simulink model "POstDeployment_ShockLoad_Calcs"  (R2022b)
settings: Solver=ode8  StartTime=0.0  StopTime=200  FixedStep=0.0001  RelTol=1e-3
values from neighbouring files (symbols this model uses):
  A_b = 0.01824    [Recovery_ShockLoad_Variables.m]
  Cdb = 0.54    [Recovery_ShockLoad_Variables.m]
  Cdp = 0.97    [Recovery_ShockLoad_Variables.m]
  g = 9.81    [Recovery_ShockLoad_Variables.m]
  mb = 38    [Recovery_ShockLoad_Variables.m]
  V_0 = 75    [Recovery_ShockLoad_Variables.m]
undefined symbols (not defined in the file or in its folder): L_m, m_m, rho, sigbuilder_block
settings Model: Creator=mohka  LastModifiedBy=mohka
settings DebuggingCC: UnconnectedInputMsg=warning  UnconnectedOutputMsg=warning  UnconnectedLineMsg=warning
settings ModelReferenceCC: EnableRefExpFcnMdlSchedulingChecks=on
settings RTWCC: DLArmComputeVersion=19.05

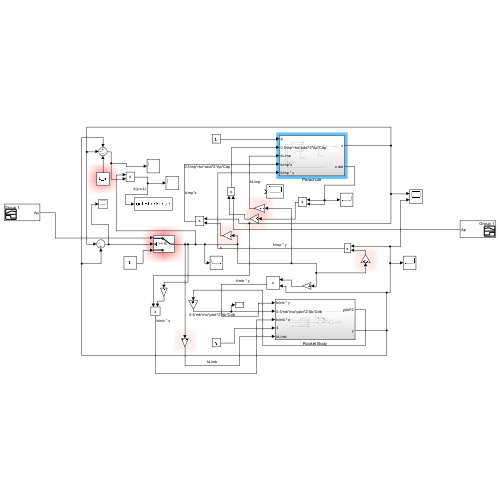
[thumbnail: Simulink's stored preview of the top-level diagram]
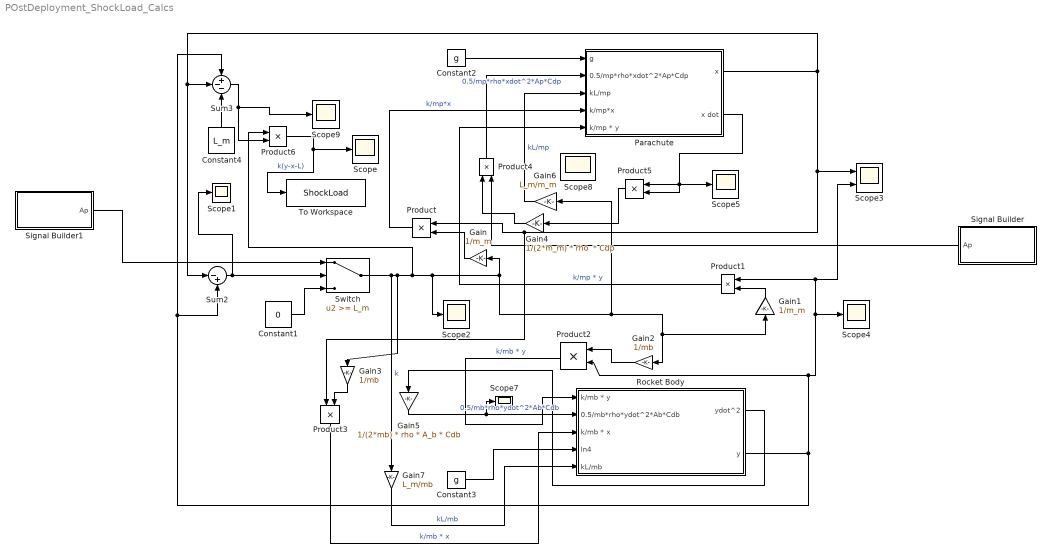
== system POstDeployment_ShockLoad_Calcs ==
  Constant1 : Constant  Value=0  VectorParams1D=off
  Constant2 : Constant  Value=g
  Constant3 : Constant  Value=g
  Constant4 : Constant  Value=L_m
  Gain : Gain  Gain=1/m_m
  Gain1 : Gain  Gain=1/m_m
  Gain2 : Gain  Gain=1/mb
  Gain3 : Gain  Gain=1/mb
  Gain4 : Gain  Gain="1/(2*m_m) * rho  * Cdp"
  Gain5 : Gain  Gain=1/(2*mb) * rho * A_b * Cdb
  Gain6 : Gain  Gain=L_m/m_m
  Gain7 : Gain  Gain=L_m/mb
  Parachute : Subsystem
  Product{,1..6} (7 alike) : Product
  Rocket Body : Subsystem
  Scope{,1..2,4..5,7..9} (8 alike) : Scope
  Scope3 : Scope  NumInputPorts=2
  Signal Builder : Subsystem  Tag=STV Subsys  LoadFcn=sigbuilder_block('load');  StartFcn=sigbuilder_block('start');  StopFcn=sigbuilder_block('stop');  ClipboardFcn=sigbuilder_block('clipboard');  mask(Sigbuilder block){tuvar=[0:10]}
      mask help: Simulink:masks:SigbuilderBlock_MD
      mask init:
      | if ~strcmp(get_param(bdroot(gcbh),'SimulationStatus'),'stopped') tuvar = sigbuilder_block('maskInit'); end
      settings: CopyFcn=sigbuilder_block('copy');  DeleteFcn=sigbuilder_block('delete');  ModelCloseFcn=sigbuilder_block('modelClose');  PreSaveFcn=sigbuilder_block('preSave');  PauseFcn=sigbuilder_block('pause');  ContinueFcn=sigbuilder_block('continue');  NameChangeFcn=sigbuilder_block('namechange');  OpenFcn=sigbuilder_block('open',[6 0 1428 711.75 ]);  CloseFcn=sigbuilder_block('close');
      mask Display: plot(0, 0, 100, 100,[2, 2, 32, 32, 2], [68, 8, 8, 68, 68],[32, 2], [38, 38], [32, 19, 2],[53, 60, 44], [32, 17, 17, 2],[16, 16, 31, 31]);txt = getActiveGroup(gcbh);text(2, 100, txt,'verticalAlignment', 'top');
  Signal Builder1 : Subsystem  Tag=STV Subsys  LoadFcn=sigbuilder_block('load');  StartFcn=sigbuilder_block('start');  StopFcn=sigbuilder_block('stop');  ClipboardFcn=sigbuilder_block('clipboard');  mask(Sigbuilder block){tuvar=[0:10]}
      mask help: Simulink:masks:SigbuilderBlock_MD
      mask init:
      | if ~strcmp(get_param(bdroot(gcbh),'SimulationStatus'),'stopped') tuvar = sigbuilder_block('maskInit'); end
      settings: CopyFcn=sigbuilder_block('copy');  DeleteFcn=sigbuilder_block('delete');  ModelCloseFcn=sigbuilder_block('modelClose');  PreSaveFcn=sigbuilder_block('preSave');  PauseFcn=sigbuilder_block('pause');  ContinueFcn=sigbuilder_block('continue');  NameChangeFcn=sigbuilder_block('namechange');  OpenFcn=sigbuilder_block('open',[116.509 88.3636 1427.56 712.145 ]);  CloseFcn=sigbuilder_block('close');
      mask Display: plot(0, 0, 100, 100,[2, 2, 32, 32, 2], [68, 8, 8, 68, 68],[32, 2], [38, 38], [32, 19, 2],[53, 60, 44], [32, 17, 17, 2],[16, 16, 31, 31]);txt = getActiveGroup(gcbh);text(2, 100, txt,'verticalAlignment', 'top');
  Sum2 : Sum  Inputs=|-+
  Sum3 : Sum  Inputs=+--
  Switch : Switch  Threshold=L_m  SaturateOnIntegerOverflow=off  InputSameDT=off
  To Workspace : ToWorkspace  VariableName=ShockLoad  SampleTime=-1
  wires:
  Gain/1 -> Product/2
  Product3/1 -> Rocket Body/3(k/mb * x)  "k/mb * x"
  Product4/1 -> Parachute/2(0.5/mp*rho*xdot^2*Ap*Cdp)  "0.5/mp*rho*xdot^2*Ap*Cdp"
  Gain7/1 -> Rocket Body/5(kL/mb)  "kL/mb"
  Product5/1 -> Gain4/1
  Rocket Body/1(ydot^2) -> Gain5/1
  Constant3/1 -> Rocket Body/4(In4)
  Constant1/1 -> Switch/3
  Parachute/2(x dot) -> Product5/1, Scope5/1, Product5/2
  Sum3/1 -> Scope9/1, Product6/2
  Product1/1 -> Parachute/5(k/mp * y)  "k/mp * y"
  Product/1 -> Parachute/4(k/mp*x)  "k/mp*x"
  Gain3/1 -> Product3/2
  Gain1/1 -> Product1/2
  Gain6/1 -> Parachute/3(kL/mp)  "kL/mp"
  Parachute/1(x) -> Product/1, Product3/1, Scope3/1, Sum2/1, Sum3/2
  Gain4/1 -> Product4/1
  Gain2/1 -> Product2/1
  Constant2/1 -> Parachute/1(g)
  Rocket Body/2(y) -> Scope3/2, Product1/1, Scope4/1, Product2/2, Sum3/1, Sum2/2
  Product6/1 -> To Workspace/1, Scope/1  "k(y-x-L)"
  Switch/1 -> Scope2/1, Gain/1, Gain6/1, Gain2/1, Gain1/1, Product6/1, Gain3/1, Gain7/1  "k"
  Gain5/1 -> Rocket Body/2(0.5/mb*rho*ydot^2*Ab*Cdb), Scope7/1  "0.5/mb*rho*ydot^2*Ab*Cdb"
  Product2/1 -> Rocket Body/1(k/mb * y)  "k/mb * y"
  Constant4/1 -> Sum3/3
  Signal Builder1/1(Ap) -> Switch/1
  Sum2/1 -> Scope1/1, Switch/2
  Signal Builder/1(Ap) -> Product4/2

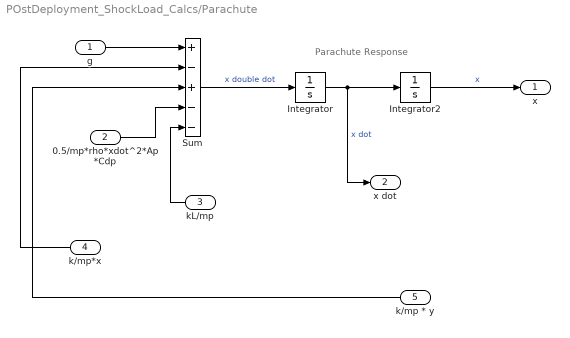
== system POstDeployment_ShockLoad_Calcs/Parachute ==
  note: Parachute Response
  g : Inport
  0.5/mp*rho*xdot^2*Ap*Cdp : Inport  Port=2
  kL/mp : Inport  Port=3
  k/mp*x : Inport  Port=4
  k/mp * y : Inport  Port=5
  Integrator : Integrator  InitialCondition=V_0
  Integrator2 : Integrator
  Sum : Sum  Inputs=+-+--
  x : Outport
  x dot : Outport  Port=2
  wires:
  Sum/1 -> Integrator/1  "x double dot"
  0.5/mp*rho*xdot^2*Ap*Cdp/1 -> Sum/4
  k/mp * y/1 -> Sum/3
  Integrator/1 -> x dot/1, Integrator2/1  "x dot"
  Integrator2/1 -> x/1  "x"
  g/1 -> Sum/1
  k/mp*x/1 -> Sum/2
  kL/mp/1 -> Sum/5

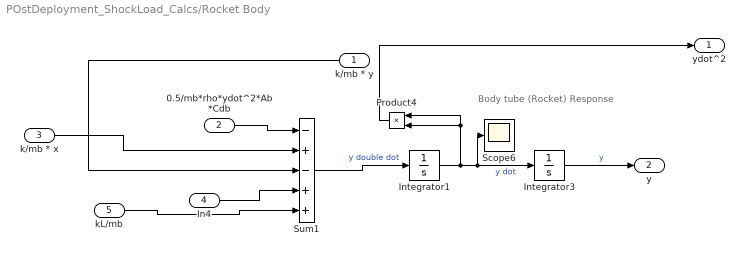
== system POstDeployment_ShockLoad_Calcs/Rocket Body ==
  note: Body tube (Rocket) Response
  k/mb * y : Inport
  0.5/mb*rho*ydot^2*Ab*Cdb : Inport  Port=2
  k/mb * x : Inport  Port=3
  In4 : Inport  Port=4
  kL/mb : Inport  Port=5
  Integrator1 : Integrator  InitialCondition=V_0
  Integrator3 : Integrator
  Product4 : Product
  Scope6 : Scope
  Sum1 : Sum  Inputs=-+-++
  ydot^2 : Outport
  y : Outport  Port=2
  wires:
  Integrator1/1 -> Scope6/1, Integrator3/1, Product4/2, Product4/1  "y dot"
  Sum1/1 -> Integrator1/1  "y double dot"
  0.5/mb*rho*ydot^2*Ab*Cdb/1 -> Sum1/1
  Integrator3/1 -> y/1  "y"
  Product4/1 -> ydot^2/1
  k/mb * y/1 -> Sum1/3
  In4/1 -> Sum1/4
  k/mb * x/1 -> Sum1/2
  kL/mb/1 -> Sum1/5

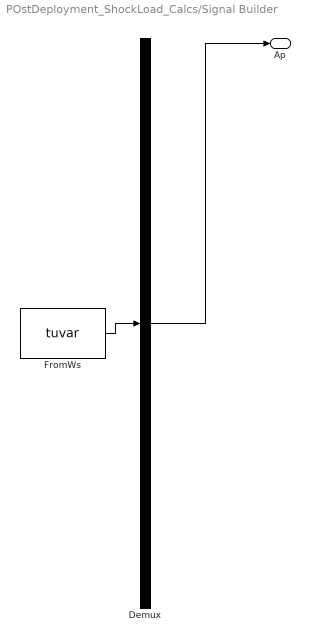
== system POstDeployment_ShockLoad_Calcs/Signal Builder ==
  Demux : Demux  Tag=STV Demux  Outputs=1
      settings: DisplayOption=none
  FromWs : FromWorkspace  Tag=STV FromWs  VariableName=tuvar
      SigBuilderData=|
      | common.afterFinalStr = 'Extrapolate'
      | common.sampleTime = 0
      | dataSet.timeRange = [0 200]
      | dataSet.name = 'Group 1'
      | sbobj.Groups.Name = 'Group 1'
      | sbobj.Groups.Signals.Name = 'Ap'
      | sbobj.Groups.Signals.XData = [0 78 78 200]
      | sbobj.Groups.Signals.YData = [0.6567 0.6567 29.1864 29.1864]
      | sbobj.Groups.TimeRange = [0 200]
  Ap : Outport  Tag=STV Outport
  wires:
  Demux/1 -> Ap/1
  FromWs/1 -> Demux/1

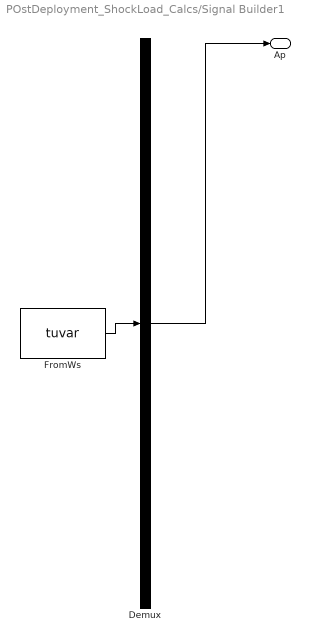
== system POstDeployment_ShockLoad_Calcs/Signal Builder1 ==
  Demux : Demux  Tag=STV Demux  Outputs=1
      settings: DisplayOption=none
  FromWs : FromWorkspace  Tag=STV FromWs  VariableName=tuvar
      SigBuilderData=|
      | common.afterFinalStr = 'Extrapolate'
      | common.sampleTime = 0
      | dataSet.timeRange = [0 200]
      | dataSet.name = 'Group 1'
      | sbobj.Groups.Name = 'Group 1'
      | sbobj.Groups.Signals.Name = 'Ap'
      | sbobj.Groups.Signals.XData = [0 78 78 200]
      | sbobj.Groups.Signals.YData = [0.6567 0.6567 29.1864 29.1864]
      | sbobj.Groups.TimeRange = [0 200]
  Ap : Outport  Tag=STV Outport
  wires:
  FromWs/1 -> Demux/1
  Demux/1 -> Ap/1
